simulink model "SF027A_EotProtnFwl"
settings: Solver=FixedStepDiscrete  SolverMode=SingleTasking  StartTime=0.0  StopTime=1  FixedStep=0.002  RelTol=1e-3
values from neighbouring files (symbols this model uses):
  ACTVREGN_CNT_U08 = DataDict.Constant    [SF027A_EotProtnFwl_DataDict.m]
  ARCHGLBPRM_FLOATZEROTHD_ULS_F32 = DataDict.Constant    [SF027A_EotProtnFwl_DataDict.m]
  EOTACTVCMDFWLREACHED_CNT_U08 = DataDict.Constant    [SF027A_EotProtnFwl_DataDict.m]
  EOTDMPGFWLREACHED_CNT_U08 = DataDict.Constant    [SF027A_EotProtnFwl_DataDict.m]
  EotProtnFwlInactvLim = DataDict.Calibration    [SF027A_EotProtnFwl_DataDict.m]
  EotProtnHwAgMin = DataDict.ImprtdCal    [SF027A_EotProtnFwl_DataDict.m]
  EotProtnHwDegDampgX = DataDict.ImprtdCal    [SF027A_EotProtnFwl_DataDict.m]
  EotProtnRackTrvlLimrRng = DataDict.ImprtdCal    [SF027A_EotProtnFwl_DataDict.m]
  EotProtnSoftEndStopAuthyThd = DataDict.ImprtdCal    [SF027A_EotProtnFwl_DataDict.m]
  FWLDISAD_CNT_U08 = DataDict.Constant    [SF027A_EotProtnFwl_DataDict.m]
  INACTVREGN_CNT_U08 = DataDict.Constant    [SF027A_EotProtnFwl_DataDict.m]
undefined symbols (not defined in the file or in its folder): MfgEnaSt1, NtcNr1, NtcSts1, sigbuilder_block
libraries: simulink x8, NxtrLim x6, FixdToFloat x5, LnrIntrpn x2, BilnrIntrpnCmnX x2, FloatToFixd x2, NxtrAbslt x1
(part 2 of 2)

== system SF027A_EotProtnFwl/EotProtnFwl/EotProtnFwlPer1/Set_Faults ==
  note: NEXTEER TROUBLE CODES
      |
      | Number                TYPE                        Name
      |  NTCNR_0X0C6      F3      NTCNumber.NTC_Num_EotProtnFwlFlt
  note: NTC Blocks
  EotDampgFwlReached : Inport  RequirementInfo={} %GIDa_fb9762c7_cb48_435d_962a_968beb3b5571
  EotActvCmdFwlReached : Inport  RequirementInfo={} %GIDa_cc26a3f8_9529_4651_9589_2e5437cfca1c  Port=2
  CopyRight2 : Subsystem  Description=|  mask(Copyright Information){none=on}
      | Copyright info block.                                               
      |                                                                     
      | Place copyright information at the top of every subsystem in design.
      mask prompts: none "No parameters"
      mask help: Place copyright information at the top of every subsystem in design.
      mask Display:
      | NxtrConf = 'Nexteer Confidential';
      | 
      | sys = bdroot; %handle for the current model ("system")
      | first = get_param(sys,'Created');
      | first = first(end-3:end);  %year is last four digits
      | 
      | last = get_param(sys,'LastModifiedDate');
      | if isempty(last)
      |     last = datestr(now,'yyyy');
      | else
      |     last = last(end-3:end);
      | end
      | 
      | if strcmp(first,last)
      |     fprintf('%s -- Copyright %s Nexteer',NxtrConf,first)
      | else
      |     fprintf('%s -- %s%s- %s Nexteer',NxtrConf,char(169),first,last)
      | end
  If : If  IfExpression=u1  ShowElse=off
  Logical Operator : Logic  Operator=OR  AllPortsSameDT=off  OutDataTypeStr=boolean
  SetEotProtnFwFlt : Subsystem  TreatAsAtomicUnit=on
  wires:
  Logical Operator/1 -> If/1
  If/1 -> SetEotProtnFwFlt/Action
  EotDampgFwlReached/1 -> SetEotProtnFwFlt/1(EotDampgFwlReached), Logical Operator/1
  EotActvCmdFwlReached/1 -> SetEotProtnFwFlt/2(EotActvCmdFwlReached), Logical Operator/2

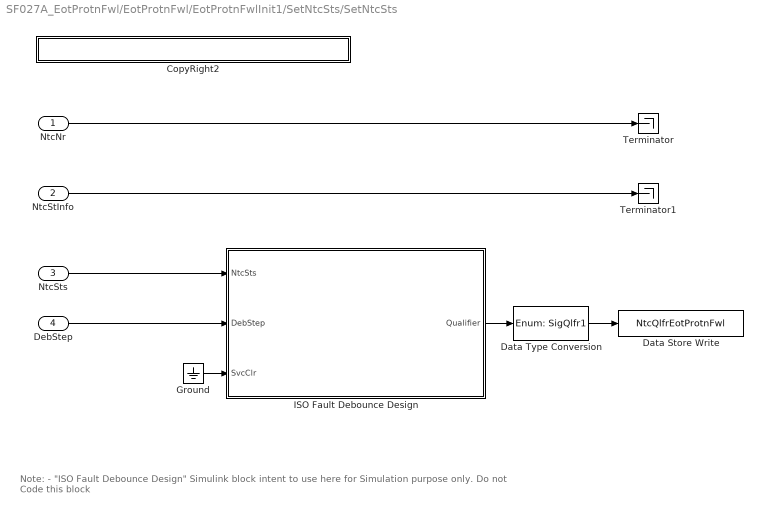
== system SF027A_EotProtnFwl/EotProtnFwl/EotProtnFwlInit1/SetNtcSts/SetNtcSts ==
  note: Note:
      |
      | - "ISO Fault Debounce Design" Simulink block intent to use here for Simulation purpose only. Do not Code this block
  NtcNr : Inport
  NtcStInfo : Inport  Port=2
  NtcSts : Inport  Port=3
  DebStep : Inport  Port=4
  CopyRight2 : Subsystem  Description=|  mask(Copyright Information){none=on}
      | Copyright info block.                                               
      |                                                                     
      | Place copyright information at the top of every subsystem in design.
      mask prompts: none "No parameters"
      mask help: Place copyright information at the top of every subsystem in design.
      mask Display:
      | NxtrConf = 'Nexteer Confidential';
      | 
      | sys = bdroot; %handle for the current model ("system")
      | first = get_param(sys,'Created');
      | first = first(end-3:end);  %year is last four digits
      | 
      | last = get_param(sys,'LastModifiedDate');
      | if isempty(last)
      |     last = datestr(now,'yyyy');
      | else
      |     last = last(end-3:end);
      | end
      | 
      | if strcmp(first,last)
      |     fprintf('%s -- Copyright %s Nexteer',NxtrConf,first)
      | else
      |     fprintf('%s -- %s%s- %s Nexteer',NxtrConf,char(169),first,last)
      | end
  Data Store Write : DataStoreWrite  DataStoreName=NtcQlfrEotProtnFwl
  Data Type Conversion : DataTypeConversion  OutDataTypeStr=Enum: SigQlfr1
  Ground : Ground
  ISO Fault Debounce Design : Stateflow chart  TreatAsAtomicUnit=on
      settings: AttributesFormatString=|
      | Simulation Purpose Only.
      | Do Not Code this block
      | Diagnostic Manager Owns this requirement
  Terminator : Terminator
  Terminator1 : Terminator
  wires:
  Data Type Conversion/1 -> Data Store Write/1
  NtcStInfo/1 -> Terminator1/1
  NtcNr/1 -> Terminator/1
  NtcSts/1 -> ISO Fault Debounce Design/1(NtcSts)
  DebStep/1 -> ISO Fault Debounce Design/2(DebStep)
  ISO Fault Debounce Design/1(Qualifier) -> Data Type Conversion/1
  Ground/1 -> ISO Fault Debounce Design/3(SvcClr)

== system SF027A_EotProtnFwl/EotProtnFwl/EotProtnFwlPer1/CalcEotActvCmdActiveRange/CopyRight2 ==

== system SF027A_EotProtnFwl/EotProtnFwl/EotProtnFwlPer1/CalcEotDampActiveRange/CopyRight2 ==

== system SF027A_EotProtnFwl/EotProtnFwl/EotProtnFwlPer1/Defeat Firewall/CopyRight2 ==

== system SF027A_EotProtnFwl/EotProtnFwl/EotProtnFwlPer1/Defeat Firewall1/CopyRight2 ==

== system SF027A_EotProtnFwl/EotProtnFwl/EotProtnFwlPer1/EotActvCmdActiveRegion/CCWCalculation ==
  CwLowrLim : Inport
  CwUpprLim : Inport  Port=2
  Action Port : ActionPort  ActionType=else
  Unary Minus1 : UnaryMinus
  Unary Minus2 : UnaryMinus
  ActvCmdLowrLim : Outport
  ActvCmdUpprLim : Outport  Port=2
  wires:
  CwUpprLim/1 -> Unary Minus2/1
  CwLowrLim/1 -> Unary Minus1/1
  Unary Minus1/1 -> ActvCmdUpprLim/1
  Unary Minus2/1 -> ActvCmdLowrLim/1

== system SF027A_EotProtnFwl/EotProtnFwl/EotProtnFwlPer1/EotActvCmdActiveRegion/CWCalculation ==
  CwLowrLim : Inport
  CwUpprLim : Inport  Port=2
  Action Port : ActionPort  ActionType=then
  ActvCmdLowrLim : Outport
  ActvCmdUpprLim : Outport  Port=2
  wires:
  CwLowrLim/1 -> ActvCmdLowrLim/1
  CwUpprLim/1 -> ActvCmdUpprLim/1

== system SF027A_EotProtnFwl/EotProtnFwl/EotProtnFwlPer1/EotActvCmdActiveRegion/CalCWLimitValues ==
  note: Calculate the CW Limit Values
  note: CCW EOT Limit values
      |                    |
      |                    |
      |                    |
      |         Y1         |
      |                    |
      |  U U U U U U U U U |
      | --------------------------------
      |                    |
      |                    |
      |                    |
      |         Y2         |
      |                    |
      |  L L L L L L L L L |
  note: CW EOT Limit values
      |                    | U U U U U U U U U U
      |                    |
      |                    |       Y2
      |                    |
      |                    |
      |                    |
      |              -------------------------------
      |                    | L L L L L L L L L L
      |                    |
      |                    |         Y1
      |                    |
      |                    |
      |                    |
  note: NOTE:
      | These tables have shared calibrations with the CW EOT direction but must be inverted and upper and lower limits swapped
      | (ie  Y1 limit for CW Lower limit becomes the CCW Upper Limit, Y2 limit for CW Upper limit becomes the CCW Lower Limit)
  VehSpd : Inport
  CopyRight2 : Subsystem  Description=|  mask(Copyright Information){none=on}
      | Copyright info block.                                               
      |                                                                     
      | Place copyright information at the top of every subsystem in design.
      mask prompts: none "No parameters"
      mask help: Place copyright information at the top of every subsystem in design.
      mask Display:
      | NxtrConf = 'Nexteer Confidential';
      | 
      | sys = bdroot; %handle for the current model ("system")
      | first = get_param(sys,'Created');
      | if(isempty(first))
      |     first = datestr(now,'yyyy');
      | else
      |     first = first(end-3:end);  %year is last four digits
      | end
      | 
      | last = get_param(sys,'LastModifiedDate');
      | if isempty(last)
      |     last = datestr(now,'yyyy');
      | else
      |     last = last(end-3:end);
      | end
      | 
      | if strcmp(first,last)
      |     fprintf('%s -- Copyright %s Nexteer',NxtrConf,first)
      | else
      |     fprintf('%s -- %s%s- %s Nexteer',NxtrConf,char(169),first,last)
      | end
  FixdToFloat_f32_s16 : FixdToFloat/FixdToFloat_f32_s16  Param1=11
  FixdToFloat_f32_s3 : FixdToFloat/FixdToFloat_f32_s16  Param1=11
  LnrIntrpn_s16_u16VariXs16VariY : LnrIntrpn/LnrIntrpn_s16_u16VariXs16VariY  XTbl=EotProtnFwlVehSpd  YTbl=EotProtnFwlActvCmdLowrBnd
      settings: AttributesFormatString=Lnr ( u16VariX , s16VariY )
  LnrIntrpn_s16_u16VariXs16VariY1 : LnrIntrpn/LnrIntrpn_s16_u16VariXs16VariY  XTbl=EotProtnFwlVehSpd  YTbl=EotProtnFwlActvCmdUpprBnd
      settings: AttributesFormatString=Lnr ( u16VariX , s16VariY )
  CwLowrLim : Outport
  CwUpprLim : Outport  Port=2
  wires:
  LnrIntrpn_s16_u16VariXs16VariY1/1 -> FixdToFloat_f32_s16/1
  LnrIntrpn_s16_u16VariXs16VariY/1 -> FixdToFloat_f32_s3/1
  FixdToFloat_f32_s16/1 -> CwUpprLim/1
  FixdToFloat_f32_s3/1 -> CwLowrLim/1
  VehSpd/1 -> LnrIntrpn_s16_u16VariXs16VariY/1, LnrIntrpn_s16_u16VariXs16VariY1/1  "VehSpd_u9p7"

== system SF027A_EotProtnFwl/EotProtnFwl/EotProtnFwlPer1/EotActvCmdActiveRegion/CopyRight2 ==

== system SF027A_EotProtnFwl/EotProtnFwl/EotProtnFwlPer1/EotActvCmdInactiveRegion/CopyRight2 ==

== system SF027A_EotProtnFwl/EotProtnFwl/EotProtnFwlPer1/EotDmpActiveRegion/CopyRight2 ==

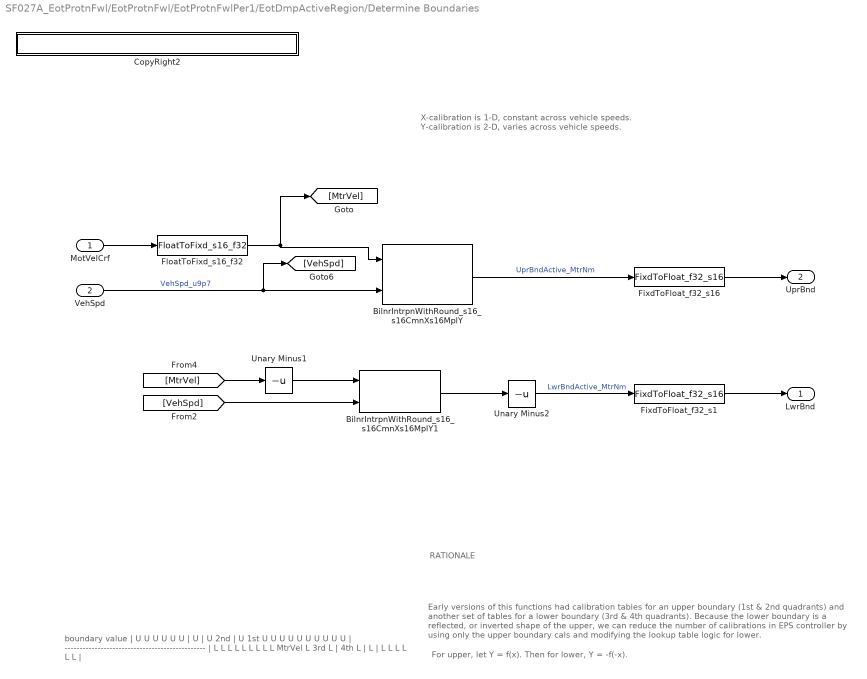
== system SF027A_EotProtnFwl/EotProtnFwl/EotProtnFwlPer1/EotDmpActiveRegion/Determine Boundaries ==
  note: boundary value
      |                    |       U U U U U U
      |                    |     U
      |                    |   U
      |       2nd          | U       1st
      |                    U
      |  U U U U U U U U U |
      | -----------------------------------------------
      |                    | L L L L L L L L L    MtrVel
      |                    L
      |       3rd        L |         4th
      |                L   |
      |              L     |
      |  L L L L L L       |
  note: RATIONALE
  note: Early versions of this functions had calibration tables for an upper boundary (1st & 2nd quadrants)
      | and another set of tables for a lower boundary (3rd & 4th quadrants).  Because the lower boundary
      | is a reflected, or inverted shape of the upper, we can reduce the number of calibrations in EPS
      | controller by using only the upper boundary cals and modifying the lookup table logic for lower.
  note: For upper, let Y = f(x). Then for lower, Y = -f(-x).
  note: X-calibration is 1-D, constant across vehicle speeds.
      | Y-calibration is 2-D, varies across vehicle speeds.
  MotVelCrf : Inport
  VehSpd : Inport  Port=2
  BilnrIntrpnWithRound_s16_s16CmnXs16MplY : BilnrIntrpnCmnX/BilnrIntrpnWithRound_s16_s16CmnXs16MplY  XTbl=EotProtnFwlEotDampgActvBndX  MplYTbl=EotProtnFwlEotDampgActvBndY  BilnrSelnTbl=EotProtnFwlVehSpd
      settings: AttributesFormatString=Bilnr ( s16CmnX , s16MplY )
  BilnrIntrpnWithRound_s16_s16CmnXs16MplY1 : BilnrIntrpnCmnX/BilnrIntrpnWithRound_s16_s16CmnXs16MplY  XTbl=EotProtnFwlEotDampgActvBndX  MplYTbl=EotProtnFwlEotDampgActvBndY  BilnrSelnTbl=EotProtnFwlVehSpd
      settings: AttributesFormatString=Bilnr ( s16CmnX , s16MplY )
  CopyRight2 : Subsystem  Description=|  mask(Copyright Information){none=on}
      | Copyright info block.                                               
      |                                                                     
      | Place copyright information at the top of every subsystem in design.
      mask prompts: none "No parameters"
      mask help: Place copyright information at the top of every subsystem in design.
      mask Display:
      | NxtrConf = 'Nexteer Confidential';
      | 
      | sys = bdroot; %handle for the current model ("system")
      | first = get_param(sys,'Created');
      | first = first(end-3:end);  %year is last four digits
      | 
      | last = get_param(sys,'LastModifiedDate');
      | if isempty(last)
      |     last = datestr(now,'yyyy');
      | else
      |     last = last(end-3:end);
      | end
      | 
      | if strcmp(first,last)
      |     fprintf('%s -- Copyright %s Nexteer',NxtrConf,first)
      | else
      |     fprintf('%s -- %s%s- %s Nexteer',NxtrConf,char(169),first,last)
      | end
  FixdToFloat_f32_s1 : FixdToFloat/FixdToFloat_f32_s16  Param1=8
  FixdToFloat_f32_s16 : FixdToFloat/FixdToFloat_f32_s16  Param1=8
  FloatToFixd_s16_f32 : FloatToFixd/FloatToFixd_s16_f32  Param1=4
  Unary Minus1 : UnaryMinus
  Unary Minus2 : UnaryMinus
  LwrBnd : Outport
  UprBnd : Outport  Port=2
  wires:
  VehSpd/1 -> [VehSpd], BilnrIntrpnWithRound_s16_s16CmnXs16MplY/2  "VehSpd_u9p7"
  BilnrIntrpnWithRound_s16_s16CmnXs16MplY1/1 -> Unary Minus2/1
  BilnrIntrpnWithRound_s16_s16CmnXs16MplY/1 -> FixdToFloat_f32_s16/1  "UprBndActive_MtrNm"
  [MtrVel] -> Unary Minus1/1
  Unary Minus2/1 -> FixdToFloat_f32_s1/1  "LwrBndActive_MtrNm"
  MotVelCrf/1 -> FloatToFixd_s16_f32/1
  FixdToFloat_f32_s16/1 -> UprBnd/1
  FixdToFloat_f32_s1/1 -> LwrBnd/1
  FloatToFixd_s16_f32/1 -> [MtrVel], BilnrIntrpnWithRound_s16_s16CmnXs16MplY/1
  Unary Minus1/1 -> BilnrIntrpnWithRound_s16_s16CmnXs16MplY1/1
  [VehSpd] -> BilnrIntrpnWithRound_s16_s16CmnXs16MplY1/2

== system SF027A_EotProtnFwl/EotProtnFwl/EotProtnFwlPer1/EotDmpInactiveRegion/CopyRight2 ==

== system SF027A_EotProtnFwl/EotProtnFwl/EotProtnFwlPer1/Set_Faults/CopyRight2 ==

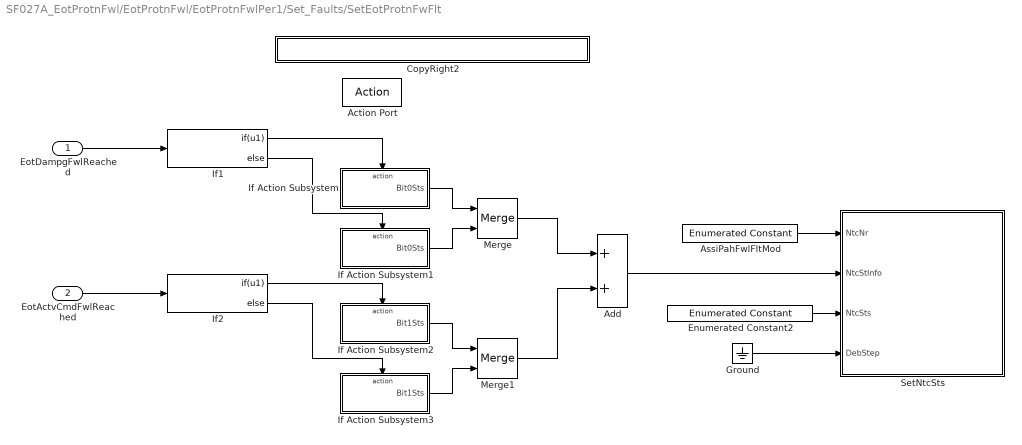
== system SF027A_EotProtnFwl/EotProtnFwl/EotProtnFwlPer1/Set_Faults/SetEotProtnFwFlt ==
  EotDampgFwlReached : Inport
  EotActvCmdFwlReached : Inport  Port=2
  Action Port : ActionPort  ActionType=then
  Add : Sum
  AssiPahFwlFltMod : simulink/Sources/Enumerated Constant  RequirementInfo={} %GIDa_cb3b210f_6485_4ea4_bbfb_6fb1b38fcd03  OutDataTypeStr=Enum: NtcNr1  Value=NtcNr1.NTCNR_0X0C6  SampleTime=inf
  CopyRight2 : Subsystem  Description=|  mask(Copyright Information){none=on}
      | Copyright info block.                                               
      |                                                                     
      | Place copyright information at the top of every subsystem in design.
      mask prompts: none "No parameters"
      mask help: Place copyright information at the top of every subsystem in design.
      mask Display:
      | NxtrConf = 'Nexteer Confidential';
      | 
      | sys = bdroot; %handle for the current model ("system")
      | first = get_param(sys,'Created');
      | first = first(end-3:end);  %year is last four digits
      | 
      | last = get_param(sys,'LastModifiedDate');
      | if isempty(last)
      |     last = datestr(now,'yyyy');
      | else
      |     last = last(end-3:end);
      | end
      | 
      | if strcmp(first,last)
      |     fprintf('%s -- Copyright %s Nexteer',NxtrConf,first)
      | else
      |     fprintf('%s -- %s%s- %s Nexteer',NxtrConf,char(169),first,last)
      | end
  Enumerated Constant2 : simulink/Sources/Enumerated Constant  RequirementInfo={} %GIDa_67cd6b05_5138_4843_bb20_7b5758eeb431  OutDataTypeStr=Enum: NtcSts1  Value=NtcSts1.NTCSTS_FAILD  SampleTime=inf
  Ground : Ground
  If Action Subsystem : Subsystem  TreatAsAtomicUnit=on
  If Action Subsystem1 : Subsystem  TreatAsAtomicUnit=on
  If Action Subsystem2 : Subsystem  TreatAsAtomicUnit=on
  If Action Subsystem3 : Subsystem  TreatAsAtomicUnit=on
  If1 : If  IfExpression=u1
  If2 : If  IfExpression=u1
  Merge : Merge
  Merge1 : Merge
  SetNtcSts : Subsystem  RequirementInfo={} %GIDa_2d43ca3c_cd6f_46db_a05f_d54808c2d2da  mask(SetNTC){}
      mask help: SetNTC library block
  wires:
  AssiPahFwlFltMod/1 -> SetNtcSts/1(NtcNr)
  Ground/1 -> SetNtcSts/4(DebStep)
  Enumerated Constant2/1 -> SetNtcSts/3(NtcSts)
  EotDampgFwlReached/1 -> If1/1
  EotActvCmdFwlReached/1 -> If2/1
  If1/1 -> If Action Subsystem/Action
  If1/2 -> If Action Subsystem1/Action
  If2/1 -> If Action Subsystem2/Action
  If2/2 -> If Action Subsystem3/Action
  Add/1 -> SetNtcSts/2(NtcStInfo)
  If Action Subsystem/1(Bit0Sts) -> Merge/1
  If Action Subsystem1/1(Bit0Sts) -> Merge/2
  If Action Subsystem2/1(Bit1Sts) -> Merge1/1
  If Action Subsystem3/1(Bit1Sts) -> Merge1/2
  Merge/1 -> Add/1
  Merge1/1 -> Add/2

== system SF027A_EotProtnFwl/EotProtnFwl/EotProtnFwlInit1/SetNtcSts/SetNtcSts/CopyRight2 ==

== system SF027A_EotProtnFwl/EotProtnFwl/EotProtnFwlPer1/EotActvCmdActiveRegion/CalCWLimitValues/CopyRight2 ==

== system SF027A_EotProtnFwl/EotProtnFwl/EotProtnFwlPer1/EotDmpActiveRegion/Determine Boundaries/CopyRight2 ==

== system SF027A_EotProtnFwl/EotProtnFwl/EotProtnFwlPer1/Set_Faults/SetEotProtnFwFlt/CopyRight2 ==

== system SF027A_EotProtnFwl/EotProtnFwl/EotProtnFwlPer1/Set_Faults/SetEotProtnFwFlt/If Action Subsystem ==
  Action Port : ActionPort  ActionType=then
  Constant : Constant  Value=EOTDMPGFWLREACHED_CNT_U08
  Constant1 : Constant  OutDataTypeStr=uint8
      settings: AttributesFormatString=%<OutDataTypeStr>
  CopyRight2 : Subsystem  Description=|  mask(Copyright Information){none=on}
      | Copyright info block.                                               
      |                                                                     
      | Place copyright information at the top of every subsystem in design.
      mask prompts: none "No parameters"
      mask help: Place copyright information at the top of every subsystem in design.
      mask Display:
      | NxtrConf = 'Nexteer Confidential';
      | 
      | sys = bdroot; %handle for the current model ("system")
      | first = get_param(sys,'Created');
      | first = first(end-3:end);  %year is last four digits
      | 
      | last = get_param(sys,'LastModifiedDate');
      | if isempty(last)
      |     last = datestr(now,'yyyy');
      | else
      |     last = last(end-3:end);
      | end
      | 
      | if strcmp(first,last)
      |     fprintf('%s -- Copyright %s Nexteer',NxtrConf,first)
      | else
      |     fprintf('%s -- %s%s- %s Nexteer',NxtrConf,char(169),first,last)
      | end
  Product1 : Product
  Bit0Sts : Outport
  wires:
  Constant/1 -> Product1/2
  Constant1/1 -> Product1/1
  Product1/1 -> Bit0Sts/1

== system SF027A_EotProtnFwl/EotProtnFwl/EotProtnFwlPer1/Set_Faults/SetEotProtnFwFlt/If Action Subsystem1 ==
  Action Port : ActionPort  ActionType=else
  Constant : Constant  Value=EOTDMPGFWLREACHED_CNT_U08
  Constant1 : Constant  Value=0  OutDataTypeStr=uint8
      settings: AttributesFormatString=%<OutDataTypeStr>
  CopyRight2 : Subsystem  Description=|  mask(Copyright Information){none=on}
      | Copyright info block.                                               
      |                                                                     
      | Place copyright information at the top of every subsystem in design.
      mask prompts: none "No parameters"
      mask help: Place copyright information at the top of every subsystem in design.
      mask Display:
      | NxtrConf = 'Nexteer Confidential';
      | 
      | sys = bdroot; %handle for the current model ("system")
      | first = get_param(sys,'Created');
      | first = first(end-3:end);  %year is last four digits
      | 
      | last = get_param(sys,'LastModifiedDate');
      | if isempty(last)
      |     last = datestr(now,'yyyy');
      | else
      |     last = last(end-3:end);
      | end
      | 
      | if strcmp(first,last)
      |     fprintf('%s -- Copyright %s Nexteer',NxtrConf,first)
      | else
      |     fprintf('%s -- %s%s- %s Nexteer',NxtrConf,char(169),first,last)
      | end
  Product1 : Product
  Bit0Sts : Outport
  wires:
  Constant/1 -> Product1/2
  Constant1/1 -> Product1/1
  Product1/1 -> Bit0Sts/1

== system SF027A_EotProtnFwl/EotProtnFwl/EotProtnFwlPer1/Set_Faults/SetEotProtnFwFlt/If Action Subsystem2 ==
  Action Port : ActionPort  ActionType=then
  Constant1 : Constant  OutDataTypeStr=uint8
      settings: AttributesFormatString=%<OutDataTypeStr>
  Constant2 : Constant  Value=EOTACTVCMDFWLREACHED_CNT_U08
  CopyRight2 : Subsystem  Description=|  mask(Copyright Information){none=on}
      | Copyright info block.                                               
      |                                                                     
      | Place copyright information at the top of every subsystem in design.
      mask prompts: none "No parameters"
      mask help: Place copyright information at the top of every subsystem in design.
      mask Display:
      | NxtrConf = 'Nexteer Confidential';
      | 
      | sys = bdroot; %handle for the current model ("system")
      | first = get_param(sys,'Created');
      | first = first(end-3:end);  %year is last four digits
      | 
      | last = get_param(sys,'LastModifiedDate');
      | if isempty(last)
      |     last = datestr(now,'yyyy');
      | else
      |     last = last(end-3:end);
      | end
      | 
      | if strcmp(first,last)
      |     fprintf('%s -- Copyright %s Nexteer',NxtrConf,first)
      | else
      |     fprintf('%s -- %s%s- %s Nexteer',NxtrConf,char(169),first,last)
      | end
  Product2 : Product
  Bit1Sts : Outport
  wires:
  Constant1/1 -> Product2/1
  Constant2/1 -> Product2/2
  Product2/1 -> Bit1Sts/1

== system SF027A_EotProtnFwl/EotProtnFwl/EotProtnFwlPer1/Set_Faults/SetEotProtnFwFlt/If Action Subsystem3 ==
  Action Port : ActionPort  ActionType=else
  Constant1 : Constant  Value=0  OutDataTypeStr=uint8
      settings: AttributesFormatString=%<OutDataTypeStr>
  Constant2 : Constant  Value=EOTACTVCMDFWLREACHED_CNT_U08
  CopyRight2 : Subsystem  Description=|  mask(Copyright Information){none=on}
      | Copyright info block.                                               
      |                                                                     
      | Place copyright information at the top of every subsystem in design.
      mask prompts: none "No parameters"
      mask help: Place copyright information at the top of every subsystem in design.
      mask Display:
      | NxtrConf = 'Nexteer Confidential';
      | 
      | sys = bdroot; %handle for the current model ("system")
      | first = get_param(sys,'Created');
      | first = first(end-3:end);  %year is last four digits
      | 
      | last = get_param(sys,'LastModifiedDate');
      | if isempty(last)
      |     last = datestr(now,'yyyy');
      | else
      |     last = last(end-3:end);
      | end
      | 
      | if strcmp(first,last)
      |     fprintf('%s -- Copyright %s Nexteer',NxtrConf,first)
      | else
      |     fprintf('%s -- %s%s- %s Nexteer',NxtrConf,char(169),first,last)
      | end
  Product2 : Product
  Bit1Sts : Outport
  wires:
  Product2/1 -> Bit1Sts/1
  Constant1/1 -> Product2/1
  Constant2/1 -> Product2/2

== system SF027A_EotProtnFwl/EotProtnFwl/EotProtnFwlPer1/Set_Faults/SetEotProtnFwFlt/SetNtcSts ==
  NtcNr : Inport
  NtcStInfo : Inport  Port=2
  NtcSts : Inport  Port=3
  DebStep : Inport  Port=4
  CopyRight2 : Subsystem  Description=|  mask(Copyright Information){none=on}
      | Copyright info block.                                               
      |                                                                     
      | Place copyright information at the top of every subsystem in design.
      mask prompts: none "No parameters"
      mask help: Place copyright information at the top of every subsystem in design.
      mask Display:
      | NxtrConf = 'Nexteer Confidential';
      | 
      | sys = bdroot; %handle for the current model ("system")
      | first = get_param(sys,'Created');
      | first = first(end-3:end);  %year is last four digits
      | 
      | last = get_param(sys,'LastModifiedDate');
      | if isempty(last)
      |     last = datestr(now,'yyyy');
      | else
      |     last = last(end-3:end);
      | end
      | 
      | if strcmp(first,last)
      |     fprintf('%s -- Copyright %s Nexteer',NxtrConf,first)
      | else
      |     fprintf('%s -- %s%s- %s Nexteer',NxtrConf,char(169),first,last)
      | end
  SetNtcSts : Subsystem  RequirementInfo={} %GIDa_724b7531_0ba9_4634_a8a7_bab8eb762083  TreatAsAtomicUnit=on
      settings: RTWSystemCode=Inline
  wires:
  NtcStInfo/1 -> SetNtcSts/2(NtcStInfo)
  DebStep/1 -> SetNtcSts/4(DebStep)
  NtcSts/1 -> SetNtcSts/3(NtcSts)
  NtcNr/1 -> SetNtcSts/1(NtcNr)  "NtcNr"

== system SF027A_EotProtnFwl/EotProtnFwl/EotProtnFwlPer1/Set_Faults/SetEotProtnFwFlt/If Action Subsystem/CopyRight2 ==

== system SF027A_EotProtnFwl/EotProtnFwl/EotProtnFwlPer1/Set_Faults/SetEotProtnFwFlt/If Action Subsystem1/CopyRight2 ==

== system SF027A_EotProtnFwl/EotProtnFwl/EotProtnFwlPer1/Set_Faults/SetEotProtnFwFlt/If Action Subsystem2/CopyRight2 ==

== system SF027A_EotProtnFwl/EotProtnFwl/EotProtnFwlPer1/Set_Faults/SetEotProtnFwFlt/If Action Subsystem3/CopyRight2 ==

== system SF027A_EotProtnFwl/EotProtnFwl/EotProtnFwlPer1/Set_Faults/SetEotProtnFwFlt/SetNtcSts/CopyRight2 ==

== system SF027A_EotProtnFwl/EotProtnFwl/EotProtnFwlPer1/Set_Faults/SetEotProtnFwFlt/SetNtcSts/SetNtcSts ==
  note: Note:
      |
      | - "ISO Fault Debounce Design" Simulink block intent to use here for Simulation purpose only. Do not Code this block
  NtcNr : Inport
  NtcStInfo : Inport  Port=2
  NtcSts : Inport  Port=3
  DebStep : Inport  Port=4
  CopyRight2 : Subsystem  Description=|  mask(Copyright Information){none=on}
      | Copyright info block.                                               
      |                                                                     
      | Place copyright information at the top of every subsystem in design.
      mask prompts: none "No parameters"
      mask help: Place copyright information at the top of every subsystem in design.
      mask Display:
      | NxtrConf = 'Nexteer Confidential';
      | 
      | sys = bdroot; %handle for the current model ("system")
      | first = get_param(sys,'Created');
      | if(isempty(first))
      |     first = datestr(now,'yyyy');
      | else
      |     first = first(end-3:end);  %year is last four digits
      | end
      | 
      | last = get_param(sys,'LastModifiedDate');
      | if isempty(last)
      |     last = datestr(now,'yyyy');
      | else
      |     last = last(end-3:end);
      | end
      | 
      | if strcmp(first,last)
      |     fprintf('%s -- Copyright %s Nexteer',NxtrConf,first)
      | else
      |     fprintf('%s -- %s%s- %s Nexteer',NxtrConf,char(169),first,last)
      | end
  Data Store Write1 : DataStoreWrite  DataStoreName=NtcQlfrEotProtnFwl
  Data Type Conversion1 : DataTypeConversion  OutDataTypeStr=Enum: SigQlfr1
  Ground : Ground
  ISO Fault Debounce Design : Stateflow chart  TreatAsAtomicUnit=on
      settings: AttributesFormatString=|
      | Simulation Purpose Only.
      | Do Not Code this block
      | Diagnostic Manager Owns this requirement
  Terminator : Terminator
  Terminator1 : Terminator
  wires:
  Ground/1 -> ISO Fault Debounce Design/3(SvcClr)
  ISO Fault Debounce Design/1(Qualifier) -> Data Type Conversion1/1
  DebStep/1 -> ISO Fault Debounce Design/2(DebStep)
  NtcNr/1 -> Terminator/1
  NtcStInfo/1 -> Terminator1/1
  NtcSts/1 -> ISO Fault Debounce Design/1(NtcSts)
  Data Type Conversion1/1 -> Data Store Write1/1

== system SF027A_EotProtnFwl/EotProtnFwl/EotProtnFwlPer1/Set_Faults/SetEotProtnFwFlt/SetNtcSts/SetNtcSts/CopyRight2 ==

== stateflow chart SF027A_EotProtnFwl/EotProtnFwl/EotProtnFwlInit1/SetNtcSts/SetNtcSts/ISO Fault Debounce Design ==
  note: NTCSTS_PASSD           (0)
      | NTCSTS_FAILD             (1)
      | NTCSTS_PREPASSD   (2)
      | NTCSTS_PREFAILD     (3)
      |
      | SIGQLFR_NORES        (0)
      | SIGQLFR_PASSD         (1)
      | SIGQLFR_FAILD           (2)
  note: Pass Loop
  note: Fail Loop
  note: 
  (default) -> (junction 89)
  (junction 89) -> (junction 95) [order 1] : [NtcSts ==3]
  (junction 89) -> (junction 93) [order 2] : [NtcSts ==2]
  (junction 89) -> (junction 141) [order 3] : [NtcSts ==1]
      | { ErrAcc = 32767;
      | Qualifier =2;
      |  }
  (junction 89) -> (junction 141) [order 4] : [NtcSts ==0]
      | { ErrAcc = -32768;
      | Qualifier=1;
      | }
  (junction 95) -> (junction 103) [order 2]
  (junction 95) -> (junction 111) [order 1] : [ErrAcc <=0]
      | {ErrAcc = DebStep;}
  (junction 93) -> (junction 123) [order 2] : {
      | ErrAcc = ErrAcc - DebStep;
      | }
  (junction 93) -> (junction 123) [order 1] : [(ErrAcc - DebStep) <= -32768]
      | { ErrAcc = -32768;
      | Qualifier=1;
      | }
  (junction 103) -> (junction 111) [order 1] : [(ErrAcc + DebStep) <32767]
      | {ErrAcc = ErrAcc + DebStep;}
  (junction 103) -> (junction 111) [order 2] : {ErrAcc = 32767;
      | Qualifier =2;}
  (junction 123) -> (junction 141)
  (junction 111) -> (junction 141)
  (junction 141) -> (junction 159) [order 2] : {ErrAcc = 0;
      | Qualifier =0;
      | }
  (junction 141) -> (junction 159) [order 1] : [SvcClr ==0]
  data: NtcSts input Enum: NtcSts1; Qualifier output uint8; DebStep input uint16; ErrAcc local single; SvcClr input

== stateflow chart SF027A_EotProtnFwl/EotProtnFwl/EotProtnFwlPer1/Set_Faults/SetEotProtnFwFlt/SetNtcSts/SetNtcSts/ISO Fault Debounce Design ==
  note: NTCSTS_PASSD           (0)
      | NTCSTS_FAILD             (1)
      | NTCSTS_PREPASSD   (2)
      | NTCSTS_PREFAILD     (3)
      |
      | SIGQLFR_NORES        (0)
      | SIGQLFR_PASSD         (1)
      | SIGQLFR_FAILD           (2)
  note: Pass Loop
  note: Fail Loop
  note: 
  (default) -> (junction 89)
  (junction 89) -> (junction 95) [order 1] : [NtcSts ==3]
  (junction 89) -> (junction 93) [order 2] : [NtcSts ==2]
  (junction 89) -> (junction 141) [order 3] : [NtcSts ==1]
      | { ErrAcc = 32767;
      | Qualifier =2;
      |  }
  (junction 89) -> (junction 141) [order 4] : [NtcSts ==0]
      | { ErrAcc = -32768;
      | Qualifier=1;
      | }
  (junction 95) -> (junction 103) [order 2]
  (junction 95) -> (junction 111) [order 1] : [ErrAcc <=0]
      | {ErrAcc = DebStep;}
  (junction 93) -> (junction 123) [order 2] : {
      | ErrAcc = ErrAcc - DebStep;
      | }
  (junction 93) -> (junction 123) [order 1] : [(ErrAcc - DebStep) <= -32768]
      | { ErrAcc = -32768;
      | Qualifier=1;
      | }
  (junction 103) -> (junction 111) [order 1] : [(ErrAcc + DebStep) <32767]
      | {ErrAcc = ErrAcc + DebStep;}
  (junction 103) -> (junction 111) [order 2] : {ErrAcc = 32767;
      | Qualifier =2;}
  (junction 123) -> (junction 141)
  (junction 111) -> (junction 141)
  (junction 141) -> (junction 159) [order 2] : {ErrAcc = 0;
      | Qualifier =0;
      | }
  (junction 141) -> (junction 159) [order 1] : [SvcClr ==0]
  data: NtcSts input Enum: NtcSts1; Qualifier output uint8; DebStep input uint16; ErrAcc local single; SvcClr input
